simulink model "Head_Light_cotrol"  (R2020a)
settings: Solver=VariableStepAuto  StartTime=0.0  StopTime=inf  RelTol=1e-3
undefined symbols (not defined in the file): DN, Light, Road_T, V_Detected
libraries: simulink x20
settings Model: Creator=VIJAY BANDEPPA MURGE  LastModifiedBy=VIJAY BANDEPPA MURGE

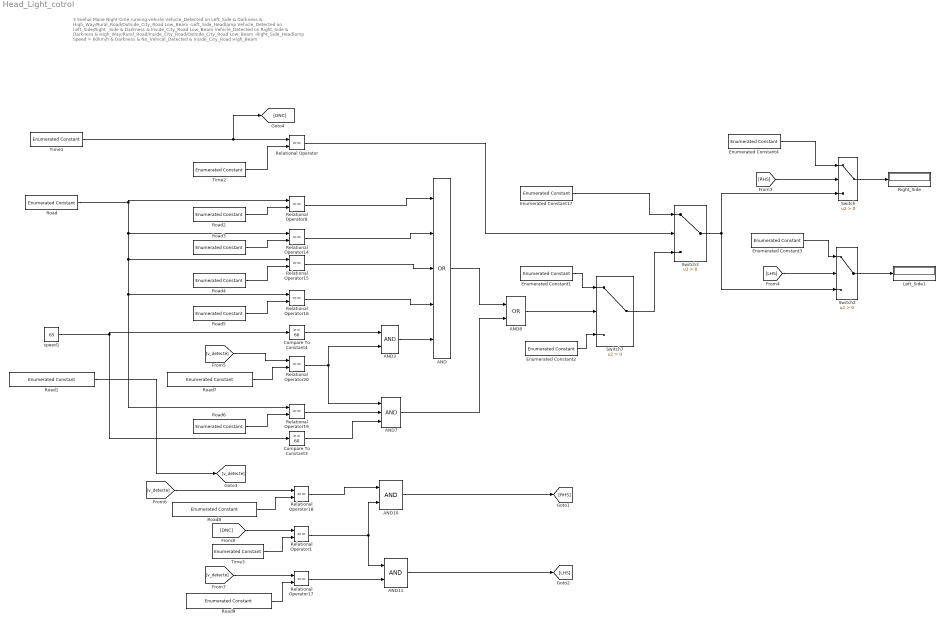
== system Head_Light_cotrol ==
  note: 3
      | Snehal Mane
      | Night-time running vehicle
      | Vehicle_Detected on Left_Side & Darkness & High_Way/Rural_Road/Outside_City_Road
      | Low_Beam -Left_Side_Headlamp
      |
      | Vehicle_Detected on Left_Side/Right _Side & Darkness & Inside_City_Road
      | Low_Beam
      |
      | Vehicle_Detected on Right_Side & Darkness & High_Way/Rural_Road/Inside_City_Road/Outside_City_Road
      | Low_Beam -Right_Side_Headlamp
      |
      | Speed > 60km/h & Darkness & No_Vehical_Detected & Inside_City_Road
      | High_Beam
  AND : Logic  Operator=OR  Inputs=5  AllPortsSameDT=off  OutDataTypeStr=boolean
  AND10 : Logic  AllPortsSameDT=off  OutDataTypeStr=boolean
  AND11 : Logic  AllPortsSameDT=off  OutDataTypeStr=boolean
  AND3 : Logic  AllPortsSameDT=off  OutDataTypeStr=boolean
  AND7 : Logic  Inputs=3  AllPortsSameDT=off  OutDataTypeStr=boolean
  AND8 : Logic  Operator=OR  AllPortsSameDT=off  OutDataTypeStr=boolean
  Compare To Constant3 : simulink/Logic and Bit Operations/Compare To Constant  relop=>=  const=60  OutDataTypeStr=boolean
  Compare To Constant4 : simulink/Logic and Bit Operations/Compare To Constant  relop=>=  const=60  OutDataTypeStr=boolean
  Enumerated Constant1 : simulink/Sources/Enumerated Constant  OutDataTypeStr=Enum: Light  Value=Light.High_beam  SampleTime=inf
  Enumerated Constant17 : simulink/Sources/Enumerated Constant  OutDataTypeStr=Enum: Light  Value=Light.Headlight_Off  SampleTime=inf
  Enumerated Constant2 : simulink/Sources/Enumerated Constant  OutDataTypeStr=Enum: Light  Value=Light.Low_Beam  SampleTime=inf
  Enumerated Constant3 : simulink/Sources/Enumerated Constant  OutDataTypeStr=Enum: Light  Value=Light.Low_Beam  SampleTime=inf
  Enumerated Constant4 : simulink/Sources/Enumerated Constant  OutDataTypeStr=Enum: Light  Value=Light.Low_Beam  SampleTime=inf
  Left_Side1 : Display
  Relational Operator{,1,8,14..20} (10 alike) : RelationalOperator  Operator===  OutDataTypeStr=boolean  RndMeth=Simplest
  Right_Side : Display
  Road : simulink/Sources/Enumerated Constant  OutDataTypeStr=Enum: Road_T  Value=Road_T.Inside_City_Road  SampleTime=inf
  Road1 : simulink/Sources/Enumerated Constant  OutDataTypeStr=Enum: V_Detected  Value=V_Detected.Vehicle_Detected_Right  SampleTime=inf
  Road2 : simulink/Sources/Enumerated Constant  OutDataTypeStr=Enum: Road_T  Value=Road_T.Express_Way  SampleTime=inf
  Road3 : simulink/Sources/Enumerated Constant  OutDataTypeStr=Enum: Road_T  Value=Road_T.High_Way  SampleTime=inf
  Road4 : simulink/Sources/Enumerated Constant  OutDataTypeStr=Enum: Road_T  Value=Road_T.Rural_Road  SampleTime=inf
  Road5 : simulink/Sources/Enumerated Constant  OutDataTypeStr=Enum: Road_T  Value=Road_T.Outside_City_Road  SampleTime=inf
  Road6 : simulink/Sources/Enumerated Constant  OutDataTypeStr=Enum: Road_T  Value=Road_T.Inside_City_Road  SampleTime=inf
  Road7 : simulink/Sources/Enumerated Constant  OutDataTypeStr=Enum: V_Detected  Value=V_Detected.No_Vehical_Detected  SampleTime=inf
  Road8 : simulink/Sources/Enumerated Constant  OutDataTypeStr=Enum: V_Detected  Value=V_Detected.Vehicle_Detected_Right  SampleTime=inf
  Road9 : simulink/Sources/Enumerated Constant  OutDataTypeStr=Enum: V_Detected  Value=V_Detected.Vehicle_Detected_Left  SampleTime=inf
  Switch{,2..3,7} (4 alike) : Switch  Criteria=u2 > Threshold
  Time1 : simulink/Sources/Enumerated Constant  OutDataTypeStr=Enum: DN  Value=DN.Darkness  SampleTime=inf
  Time2 : simulink/Sources/Enumerated Constant  OutDataTypeStr=Enum: DN  Value=DN.Day_Time  SampleTime=inf
  Time3 : simulink/Sources/Enumerated Constant  OutDataTypeStr=Enum: DN  Value=DN.Darkness  SampleTime=inf
  speed1 : Constant  Value=65
  wires:
  Enumerated Constant4/1 -> Switch/1
  Switch2/1 -> Left_Side1/1
  AND8/1 -> Switch7/2
  Switch/1 -> Right_Side/1
  Relational Operator20/1 -> AND7/1, AND3/2
  Enumerated Constant1/1 -> Switch7/1
  Relational Operator15/1 -> AND/3
  Road1/1 -> [v_detecte]
  Enumerated Constant3/1 -> Switch2/1
  Road/1 -> Relational Operator8/1, Relational Operator19/1, Relational Operator16/1, Relational Operator15/1, Relational Operator14/1
  Switch3/1 -> Switch/3, Switch2/3
  Road2/1 -> Relational Operator8/2
  Road4/1 -> Relational Operator15/2
  Time1/1 -> [DNC], Relational Operator/1
  Road7/1 -> Relational Operator20/2
  Road6/1 -> Relational Operator19/2
  Relational Operator8/1 -> AND/1
  Compare To Constant3/1 -> AND7/3
  AND/1 -> AND8/1
  AND3/1 -> AND/5
  Enumerated Constant17/1 -> Switch3/1
  Relational Operator14/1 -> AND/2
  Switch7/1 -> Switch3/3
  Relational Operator16/1 -> AND/4
  Compare To Constant4/1 -> AND3/1
  Road5/1 -> Relational Operator16/2
  Road3/1 -> Relational Operator14/2
  Enumerated Constant2/1 -> Switch7/3
  Road9/1 -> Relational Operator17/2
  Relational Operator18/1 -> AND10/1
  AND7/1 -> AND8/2
  Relational Operator19/1 -> AND7/2
  speed1/1 -> Compare To Constant3/1, Compare To Constant4/1
  Relational Operator/1 -> Switch3/2
  AND10/1 -> [RHS]
  [RHS] -> Switch/2
  AND11/1 -> [LHS]
  [LHS] -> Switch2/2
  [v_detecte] -> Relational Operator17/1
  [v_detecte] -> Relational Operator18/1
  [v_detecte] -> Relational Operator20/1
  Time2/1 -> Relational Operator/2
  Road8/1 -> Relational Operator18/2
  [DNC] -> Relational Operator1/1
  Time3/1 -> Relational Operator1/2
  Relational Operator1/1 -> AND11/1, AND10/2
  Relational Operator17/1 -> AND11/2
